simulink model "svpwm_keshav"  (R2023b)
settings: Solver=ode23t  StartTime=0.0  StopTime=0.1  MaxStep=1e-6  RelTol=1e-3
libraries: simulink x4
settings Model: Creator=ixale  LastModifiedBy=ixale

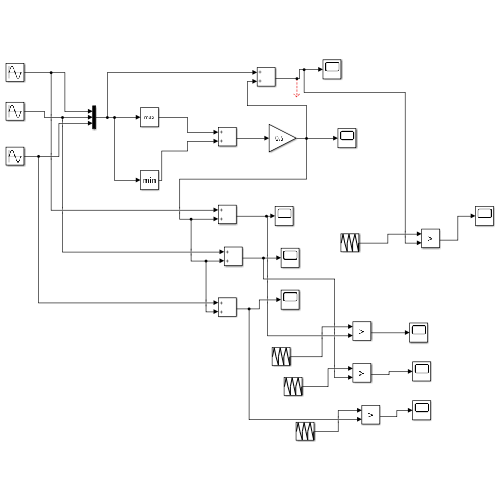
[thumbnail: Simulink's stored preview of the top-level diagram]
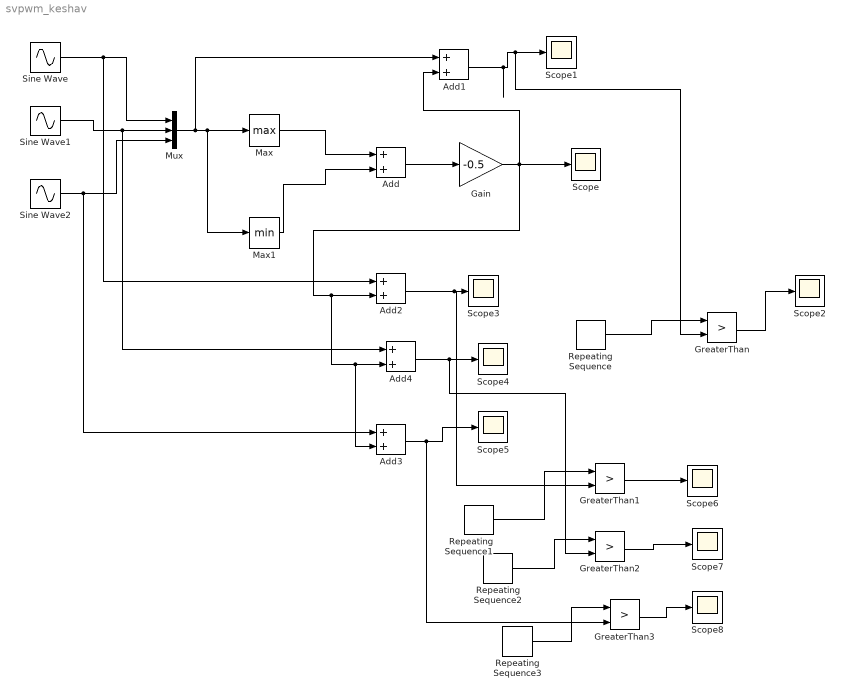
== system svpwm_keshav ==
  Add{,1..4} (5 alike) : Sum
  Gain : Gain  Gain=-0.5
  GreaterThan{,1..3} (4 alike) : RelationalOperator  Operator=>  OutDataTypeStr=boolean  RndMeth=Simplest  InputSameDT=off
  Max : MinMax  Function=max
  Max1 : MinMax
  Mux : Mux  Inputs=3
  Repeating Sequence{,1..3} (4 alike) : simulink/Sources/Repeating Sequence  rep_seq_t=[0 1 2 3]/2000  rep_seq_y=[0 1 0 -1]
  Scope{,1..8} (9 alike) : Scope
  Sine Wave : Sin  Frequency=2*pi*50  SampleTime=0
  Sine Wave1 : Sin  Frequency=2*pi*50  Phase=-2*pi/3  SampleTime=0
  Sine Wave2 : Sin  Frequency=2*pi*50  Phase=2*pi/3  SampleTime=0
  wires:
  Sine Wave/1 -> Add2/1, Mux/1
  Sine Wave1/1 -> Add4/1, Mux/2
  Sine Wave2/1 -> Add3/1, Mux/3
  Mux/1 -> Add1/1, Max1/1, Max/1
  Max/1 -> Add/1
  Max1/1 -> Add/2
  Add/1 -> Gain/1
  Gain/1 -> Add3/2, Add4/2, Add2/2, Add1/2, Scope/1
  Add1/1 -> GreaterThan/2, Scope1/1
  Repeating Sequence/1 -> GreaterThan/1
  GreaterThan/1 -> Scope2/1
  Add2/1 -> GreaterThan1/2, Scope3/1
  Add4/1 -> GreaterThan2/2, Scope4/1
  Add3/1 -> GreaterThan3/2, Scope5/1
  Repeating Sequence1/1 -> GreaterThan1/1
  Repeating Sequence2/1 -> GreaterThan2/1
  Repeating Sequence3/1 -> GreaterThan3/1
  GreaterThan1/1 -> Scope6/1
  GreaterThan2/1 -> Scope7/1
  GreaterThan3/1 -> Scope8/1
